simulink model "quadrotor_6dof_lqr"  (R2024b)
settings: Solver=FixedStepAuto  StartTime=0.0  StopTime=15  FixedStep=0.01  RelTol=1e-3
settings Model: Creator=Trey  LastModifiedBy=Trey

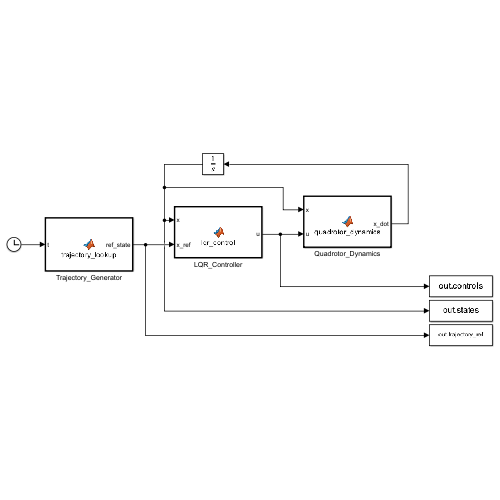
[thumbnail: Simulink's stored preview of the top-level diagram]
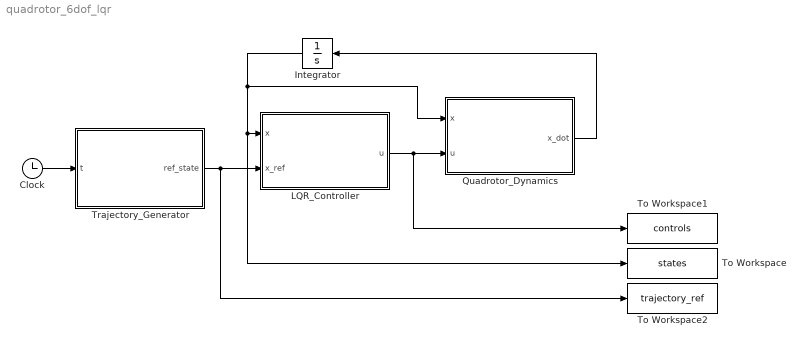
== system quadrotor_6dof_lqr ==
  Clock : Clock
  Integrator : Integrator  InitialCondition=[0;0;0;0;0;0;0;0;0;0;0;0]
  LQR_Controller : MATLAB Function  TreatAsAtomicUnit=on
  Quadrotor_Dynamics : MATLAB Function  TreatAsAtomicUnit=on
  To Workspace : ToWorkspace  VariableName=states  SaveFormat=Timeseries  SampleTime=-1
  To Workspace1 : ToWorkspace  VariableName=controls  SaveFormat=Timeseries  SampleTime=-1
  To Workspace2 : ToWorkspace  VariableName=trajectory_ref  SaveFormat=Timeseries  SampleTime=-1
  Trajectory_Generator : MATLAB Function  TreatAsAtomicUnit=on
  wires:
  Trajectory_Generator/1(ref_state) -> To Workspace2/1, LQR_Controller/2(x_ref)
  LQR_Controller/1(u) -> To Workspace1/1, Quadrotor_Dynamics/2(u)
  Clock/1 -> Trajectory_Generator/1(t)
  Quadrotor_Dynamics/1(x_dot) -> Integrator/1
  Integrator/1 -> To Workspace/1, LQR_Controller/1(x), Quadrotor_Dynamics/1(x)

== matlab function quadrotor_6dof_lqr/Trajectory_Generator ==
  data: t input; ref_state output
function ref_state = trajectory_lookup(t)
% inputs
% t: time

% outputs
% ref_state: 12x1

    persistent traj
    if isempty(traj)
        traj = evalin('base', 'trajectory');
    end
    
    % Interpolate trajectory at current time
    idx = min(max(1, round(t/traj.dt) + 1), length(traj.time));
    
    ref_state = zeros(12,1);
    ref_state(1:3) = traj.pos(idx,:)';      % Position
    ref_state(4) = traj.phi_d(idx);         % Roll
    ref_state(5) = traj.theta_d(idx);       % Pitch
    ref_state(6) = traj.yaw(idx);           % Yaw
    ref_state(7:9) = traj.vel(idx,:)';      % Velocity
    ref_state(12) = traj.yaw_rate(idx);     % Yaw rate
end

== matlab function quadrotor_6dof_lqr/Quadrotor_Dynamics ==
  data: x input; u input; x_dot output
function x_dot = quadrotor_dynamics(x, u)
% inputs
% x: state, 12x1
% u: control, 4x1

% outputs
% x_dot: state rate of change, 12x1

    persistent m g Ixx Iyy Izz
    if isempty(m)
        params = evalin('base', 'params');
        m = params.m;
        g = params.g;
        Ixx = params.Ixx;
        Iyy = params.Iyy;
        Izz = params.Izz;
    end
    
    % Parse state
    phi = x(4); theta = x(5); psi = x(6);
    v = x(7:9);
    omega = x(10:12);
    
    % Parse control
    F = u(1);
    tau = u(2:4);
    
    % Rotation matrix (body to inertial)
    R = [cos(psi)*cos(theta), cos(psi)*sin(theta)*sin(phi) - sin(psi)*cos(phi), ...
         cos(psi)*sin(theta)*cos(phi) + sin(psi)*sin(phi);
         sin(psi)*cos(theta), sin(psi)*sin(theta)*sin(phi) + cos(psi)*cos(phi), ...
         sin(psi)*sin(theta)*cos(phi) - cos(psi)*sin(phi);
         -sin(theta), cos(theta)*sin(phi), cos(theta)*cos(phi)];
    
    % Angular velocity transformation
    W = [1, sin(phi)*tan(theta), cos(phi)*tan(theta);
         0, cos(phi), -sin(phi);
         0, sin(phi)/cos(theta), cos(phi)/cos(theta)];
    
    % State derivatives
    x_dot = zeros(12,1);
    
    % Position derivative = velocity
    x_dot(1:3) = v;
    
    % Attitude derivative
    x_dot(4:6) = W * omega;
    
    % Velocity derivative (Newton's 2nd law)
    thrust_inertial = R * [0; 0; F];
    gravity = [0; 0; -m*g];
    x_dot(7:9) = (thrust_inertial + gravity) / m;
    
    % Angular acceleration (Euler's equations)
    x_dot(10) = (tau(1) - (Izz - Iyy)*omega(2)*omega(3)) / Ixx;
    x_dot(11) = (tau(2) - (Ixx - Izz)*omega(1)*omega(3)) / Iyy;
    x_dot(12) = (tau(3) - (Iyy - Ixx)*omega(1)*omega(2)) / Izz;
end

== matlab function quadrotor_6dof_lqr/LQR_Controller ==
  data: x input; u output; x_ref input
function u = lqr_control(x, x_ref)
% inputs
% x: current state, 12x1
% x_ref: reference state, 12x1

% outputs
% u: control, 4x1

    persistent K u_hover
    if isempty(K)
        params = evalin('base', 'params');
        K = params.K;
        u_hover = params.u_hover;
    end
    
    % State error
    e = x - x_ref;
    
    % LQR control law
    u = u_hover - K * e;
    
    % Saturate controls
    u(1) = max(0, min(15, u(1)));      % Thrust: 0-15 N
    u(2:4) = max(-1, min(1, u(2:4)));  % Torques: ±1 N·m
end
